simulink model "TwoArea_MA_FixedWM"  (R2020b)
settings: Solver=ode3  StartTime=0.0  StopTime=t  FixedStep=0.01  RelTol=1e-3
values from neighbouring files (symbols this model uses):
  AGC_midway = 0    [TwoAreaAGC_Parameters_Start_MA.m]    (also in result_agcimprovement.m = 1; result_replayimpact.m; result_replayimpactvaryingload.m; result_replaywithoutwm.m)
  Apc = [-par.D/(2*par.H)  1/(2*par.H)  0  -1/(2*par.H) ... (first row only)    [get_ssplant_1turb.m]
  Aq = zeros(N,N,nyp)    [offline_watermarking.m]
  attack_cont = 1    [TwoAreaAGC_Parameters_Start_MA.m]    (also in result_agcimprovement.m = 0; result_replayimpact.m; result_replayimpactvaryingload.m = 0; result_replaywithoutwm.m)
  attack_meas = 1    [TwoAreaAGC_Parameters_Start_MA.m]    (also in result_agcimprovement.m = 0; result_replayimpact.m; result_replayimpactvaryingload.m; result_replaywithoutwm.m)
  attack_start = 300    [TwoAreaAGC_Parameters_Start_MA.m]
  attack_type = 1    [TwoAreaAGC_Parameters_Start_MA.m]    (also in result_agcimprovement.m; result_replayimpact.m; result_replayimpactvaryingload.m; result_replaywithoutwm.m)
  Aw = zeros(N,N,nyp)    [offline_watermarking.m]
  Bpc = [0  -1/(2*par.H) ... (first row only)    [get_ssplant_1turb.m]
  Bq = zeros(N,1,nyp)    [offline_watermarking.m]
  Bw = zeros(N,1,nyp)    [offline_watermarking.m]
  C_sysd = c2d(C_sysc,ts_c)    [get_sscontr_2area.m]
  Cpc = [1 0 0 0 ... (first row only)    [get_ssplant_1turb.m]
  Cq = zeros(1,N,nyp)    [offline_watermarking.m]
  Cw = zeros(1,N,nyp)    [offline_watermarking.m]
  Dq = zeros(1,1,nyp)    [offline_watermarking.m]
  Dw = zeros(1,1,nyp)    [offline_watermarking.m]
  Ps = 2    [TwoAreaAGC_Parameters_Start_MA.m]
  scaling_replay = 2    [TwoAreaAGC_Parameters_Start_MA.m]    (also in result_agcimprovement.m = 1; result_replayimpact.m; result_replayimpactvaryingload.m; result_replaywithoutwm.m)
  status_load = 0    [TwoAreaAGC_Parameters_Start_MA.m]    (also in result_agcimprovement.m; result_replayimpact.m; result_replayimpactvaryingload.m = 1; result_replaywithoutwm.m)
  status_wm = 1    [TwoAreaAGC_Parameters_Start_MA.m]    (also in result_agcimprovement.m = 0; result_replayimpact.m = 0; result_replayimpactvaryingload.m = 0; result_replaywithoutwm.m = 0)
  ts = 1e-2    (= 0.01)    [TwoAreaAGC_Parameters_Start_MA.m]
undefined symbols (not defined in the file or in its folder): Ag, Ah, Bg, Bh, ca, Cg, Ch, Dg, Dh, DiscIntNeverNeededParam, Dpc, eta1, eta2, L1, L2, obs1, obs2, P1_sysd, P2_sysd, par1, par2, wm, xi1, xi2
libraries: cstblocks x16, dspsrcs4 x5, eeLuenbergerObserver x2
(part 1 of 2)
settings Model: Creator=HP  LastModifiedBy=gvandenbroek
settings DataIOCC: ReturnWorkspaceOutputs=off
settings DebuggingCC: ArithmeticOperatorsInVariantConditions=warning
settings SFSimCC: SimUseLocalCustomCode=off  CustomCodeUndefinedFunction=UseInterfaceOnly
settings RTWCC: RTWUseLocalCustomCode=off
settings CodeAppCC: StateflowObjectComments=on
settings ConfigComp: PLC_TargetIDE=twincat3

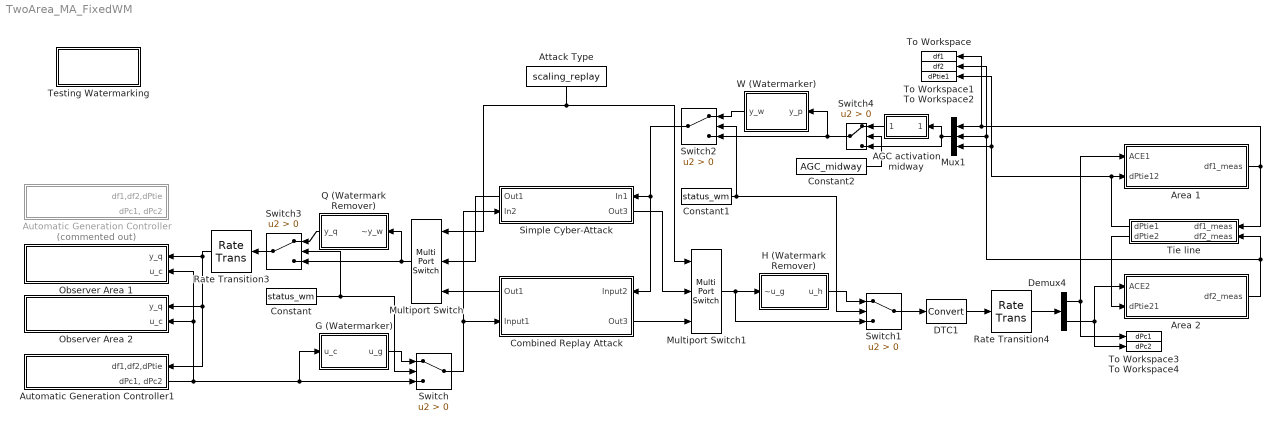
== system TwoArea_MA_FixedWM ==
  AGC activation midway : Subsystem
  Area 1 : Subsystem
  Area 2 : Subsystem
  Attack Type : Constant  Value=scaling_replay
  Automatic Generation Controller : Subsystem  Commented=on  TreatAsAtomicUnit=on
      settings: PortSchema="{\"entries\":[{\"content\":{\"sides\":[{\"content\":{\"connectorIds\":[]},\"type\":\"ConnectorPlacement.EquallySpacedRectSide\",\"uuid\":\"5549200c-2470-4b9f-b5b6-404335018806\"},{\"content\":{\"connectorIds\":[\"In1\",\"Out1\"],\"side\":\"RIGHT\"},\"type\":\"ConnectorPlacement.EquallySpacedRectSide\",\"uuid\":\"92a60021-22f8-453b-8267-494e0677e7ef\"},{\"content\":{\"connectorIds\":[],\"side\":\"TOP\"},\"type\":\"ConnectorPlacement.EquallySpacedRectSide\",\"uuid\":\"846800f7-206a-46ef-bf7f-e65eb2b7ee13\"}]},\"type\":\"ConnectorPlacement.EquallySpacedConnector\",\"uuid\":\"849222ff-13db-4c5e-adb1-95e3c523a6ec\"}],\"packageUris\":[\"http://schema.mathworks.com/mf0/Connector/19700101\"],\"version\":\"1.0\"}"
  Automatic Generation Controller1 : Subsystem  TreatAsAtomicUnit=on
      settings: PortSchema="{\"entries\":[{\"content\":{\"sides\":[{\"content\":{\"connectorIds\":[]},\"type\":\"ConnectorPlacement.EquallySpacedRectSide\",\"uuid\":\"5549200c-2470-4b9f-b5b6-404335018806\"},{\"content\":{\"connectorIds\":[\"In1\",\"Out1\"],\"side\":\"RIGHT\"},\"type\":\"ConnectorPlacement.EquallySpacedRectSide\",\"uuid\":\"92a60021-22f8-453b-8267-494e0677e7ef\"},{\"content\":{\"connectorIds\":[],\"side\":\"TOP\"},\"type\":\"ConnectorPlacement.EquallySpacedRectSide\",\"uuid\":\"846800f7-206a-46ef-bf7f-e65eb2b7ee13\"}]},\"type\":\"ConnectorPlacement.EquallySpacedConnector\",\"uuid\":\"849222ff-13db-4c5e-adb1-95e3c523a6ec\"}],\"packageUris\":[\"http://schema.mathworks.com/mf0/Connector/R2020b\"],\"version\":\"1.0\"}"
  Combined Replay Attack : Subsystem
      settings: PortSchema="{\"entries\":[{\"content\":{\"sides\":[{\"content\":{\"connectorIds\":[\"In1\",\"Out2\"]},\"type\":\"ConnectorPlacement.EquallySpacedRectSide\",\"uuid\":\"ed098d6b-24bb-4b63-8622-61583d169173\"},{\"content\":{\"connectorIds\":[\"Out1\",\"In2\"],\"side\":\"RIGHT\"},\"type\":\"ConnectorPlacement.EquallySpacedRectSide\",\"uuid\":\"5227fdb7-d0b7-460e-b294-cace27174690\"},{\"content\":{\"connectorIds\":[],\"side\":\"TOP\"},\"type\":\"ConnectorPlacement.EquallySpacedRectSide\",\"uuid\":\"40035942-24d6-4e32-87fb-1400cccdfaf4\"},{\"content\":{\"connectorIds\":[],\"side\":\"HIDDEN\"},\"type\":\"ConnectorPlacement.EquallySpacedRectSide\",\"uuid\":\"cfa004c0-44dd-4a73-bda5-a763349795eb\"}]},\"type\":\"ConnectorPlacement.EquallySpacedConnector\",\"uuid\":\"e601dc09-6e07-4799-9690-340a3e9b8374\"}],\"packageUris\":[\"http://schema.mathworks.com/mf0/Connector/R2020b\"],\"version\":\"1.0\"}"
  Constant : Constant  Value=status_wm
  Constant1 : Constant  Value=status_wm
  Constant2 : Constant  Value=AGC_midway
  DTC1 : DataTypeConversion
  Demux4 : Demux  Outputs=2
  G (Watermarker) : Subsystem
  H (Watermark Remover) : Subsystem
  Multiport Switch : MultiPortSwitch  DataPortOrder=Specify indices  DataPortIndices={1,2}
  Multiport Switch1 : MultiPortSwitch  DataPortOrder=Specify indices  DataPortIndices={1,2}
  Mux1 : Mux  Inputs=3
  Observer Area 1 : Subsystem
  Observer Area 2 : Subsystem
  Q (Watermark Remover) : Subsystem
  Rate Transition3 : RateTransition  OutPortSampleTime=ts
  Rate Transition4 : RateTransition  Integrity=off  InitialCondition=1.6  OutPortSampleTime=0
  Simple Cyber-Attack : Subsystem
      settings: PortSchema="{\"entries\":[{\"content\":{\"sides\":[{\"content\":{\"connectorIds\":[\"In1\",\"Out2\"]},\"type\":\"ConnectorPlacement.EquallySpacedRectSide\",\"uuid\":\"2958ed8f-b955-4611-80df-9c2e2faeeed8\"},{\"content\":{\"connectorIds\":[\"Out1\",\"In2\"],\"side\":\"RIGHT\"},\"type\":\"ConnectorPlacement.EquallySpacedRectSide\",\"uuid\":\"bb242c12-8aed-4e93-92e3-aa1a58434ea1\"},{\"content\":{\"connectorIds\":[],\"side\":\"TOP\"},\"type\":\"ConnectorPlacement.EquallySpacedRectSide\",\"uuid\":\"026445f8-91a1-47c1-afd6-e1ddb7405b1a\"},{\"content\":{\"connectorIds\":[],\"side\":\"BOTTOM\"},\"type\":\"ConnectorPlacement.EquallySpacedRectSide\",\"uuid\":\"f5ef18f8-9aaf-4c82-8169-2595013f0f61\"}]},\"type\":\"ConnectorPlacement.EquallySpacedConnector\",\"uuid\":\"16e2adc2-f66f-41a6-a84c-2e0eb9d1d8a6\"}],\"packageUris\":[\"http://schema.mathworks.com/mf0/Connector/19700101\"],\"version\":\"1.0\"}"
  Switch{,1..4} (5 alike) : Switch  Criteria=u2 > Threshold
  Testing Watermarking : Subsystem
  Tie line : Subsystem
  To Workspace : ToWorkspace  VariableName=df1  SampleTime=ts
  To Workspace1 : ToWorkspace  VariableName=df2  SampleTime=ts
  To Workspace2 : ToWorkspace  VariableName=dPtie1  SampleTime=ts
  To Workspace3 : ToWorkspace  VariableName=dPc1  SampleTime=ts
  To Workspace4 : ToWorkspace  VariableName=dPc2  SampleTime=ts
  W (Watermarker) : Subsystem  TreatAsAtomicUnit=on
  wires:
  Attack Type/1 -> Multiport Switch1/1, Multiport Switch/1
  Simple Cyber-Attack/1(Out1) -> Multiport Switch/2
  Switch3/1 -> Rate Transition3/1
  DTC1/1 -> Rate Transition4/1
  Multiport Switch/1 -> Switch3/3, Q (Watermark Remover)/1(~y_w)
  W (Watermarker)/1(y_w) -> Switch2/1
  Switch2/1 -> Combined Replay Attack/1(Input2), Simple Cyber-Attack/1(In1)
  Rate Transition3/1 -> Automatic Generation Controller1/1(df1,df2,dPtie), Observer Area 2/1(y_q), Observer Area 1/1(y_q)
  Q (Watermark Remover)/1(y_q) -> Switch3/1
  Simple Cyber-Attack/2(Out3) -> Multiport Switch1/2
  H (Watermark Remover)/1(u_h) -> Switch1/1
  Switch/1 -> Simple Cyber-Attack/2(In2), Combined Replay Attack/2(Input1)
  G (Watermarker)/1(u_g) -> Switch/1
  Switch1/1 -> DTC1/1
  Multiport Switch1/1 -> Switch1/3, H (Watermark Remover)/1(~u_g)
  Area 1/1(df1_meas) -> To Workspace/1, Mux1/1, Tie line/1(df1_meas)
  Area 2/1(df2_meas) -> To Workspace1/1, Mux1/2, Tie line/2(df2_meas)
  Tie line/2(dPtie2) -> Area 2/2(dPtie21)
  Tie line/1(dPtie1) -> To Workspace2/1, Mux1/3, Area 1/2(dPtie12)
  Automatic Generation Controller1/1("dPc1, dPc2") -> Observer Area 2/2(u_c), Observer Area 1/2(u_c), Switch/3, G (Watermarker)/1(u_c)
  Demux4/1 -> To Workspace3/1, Area 1/1(ACE1)
  Demux4/2 -> To Workspace4/1, Area 2/1(ACE2)
  Rate Transition4/1 -> Demux4/1
  Switch4/1 -> Switch2/3, W (Watermarker)/1(y_p)
  Constant/1 -> Switch/2, Switch3/2
  Constant1/1 -> Switch2/2, Switch1/2
  AGC activation midway/1(Out1) -> Switch4/1
  Mux1/1 -> Switch4/3, AGC activation midway/1(In1)
  Constant2/1 -> Switch4/2
  Combined Replay Attack/1(Out1) -> Multiport Switch/3
  Combined Replay Attack/2(Out3) -> Multiport Switch1/3

== system TwoArea_MA_FixedWM/AGC activation midway ==
  In1 : Inport
  Clock : Clock
  Constant : Constant  Value=0
  Demux : Demux  Outputs=3
  Mux : Mux  Inputs=3
  Switch : Switch  Threshold=attack_start
  Switch1 : Switch  Threshold=attack_start
  Switch2 : Switch  Threshold=attack_start
  Out1 : Outport
  wires:
  Switch/1 -> Mux/1
  Clock/1 -> Switch2/2, Switch1/2, Switch/2
  Demux/1 -> Switch/1
  Constant/1 -> Switch2/3, Switch1/3, Switch/3
  Demux/2 -> Switch1/1
  Switch1/1 -> Mux/2
  Demux/3 -> Switch2/1
  Switch2/1 -> Mux/3
  Mux/1 -> Out1/1
  In1/1 -> Demux/1

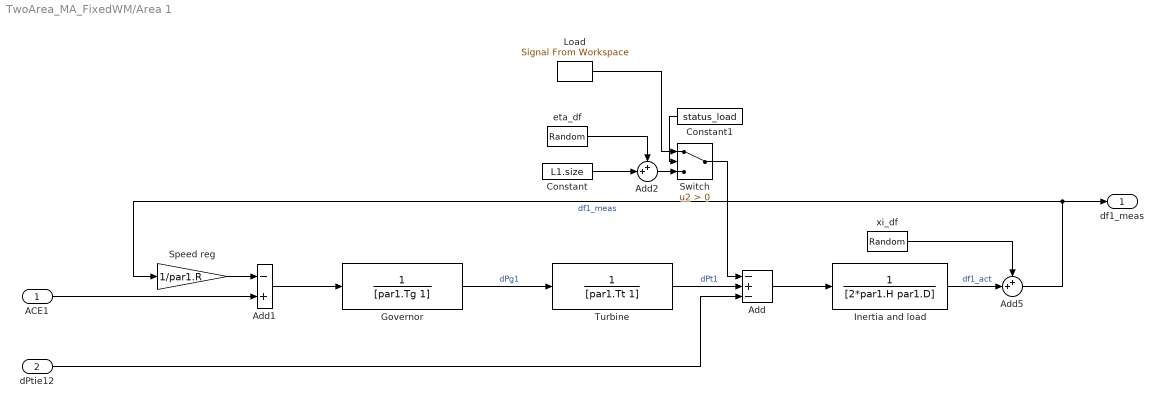
== system TwoArea_MA_FixedWM/Area 1 ==
  ACE1 : Inport
  dPtie12 : Inport  Port=2
  Add : Sum  Inputs=-+-
  Add1 : Sum  Inputs=-+
  Add2 : Sum  Inputs=++|
  Add5 : Sum  Inputs=++|
  Constant : Constant  Value=L1.size
  Constant1 : Constant  Value=status_load
  Governor : TransferFcn  Denominator=[par1.Tg 1]
  Inertia and load : TransferFcn  Denominator=[2*par1.H par1.D]
  Load : dspsrcs4/Signal From Workspace  X=L1.seq  Ts=1  nsamps=1  OutputAfterFinalValue=Holding final value  ignoreOrWarnInputAndFrameLengths=off  OutputFrames=off
  Speed reg : Gain  Gain=1/par1.R
  Switch : Switch  Criteria=u2 > Threshold
  Turbine : TransferFcn  Denominator=[par1.Tt 1]
  eta_df : RandomNumber  Variance=eta1.var(1)  Seed=eta1.seeddf  SampleTime=0
  xi_df : RandomNumber  Variance=xi1.var(1)  Seed=xi1.seeddf  SampleTime=0
  df1_meas : Outport
  wires:
  xi_df/1 -> Add5/1
  Add/1 -> Inertia and load/1
  Governor/1 -> Turbine/1  "dPg1"
  Turbine/1 -> Add/2  "dPt1"
  ACE1/1 -> Add1/2
  Add5/1 -> Speed reg/1, df1_meas/1  "df1_meas"
  Add1/1 -> Governor/1
  Inertia and load/1 -> Add5/2  "df1_act"
  Speed reg/1 -> Add1/1
  dPtie12/1 -> Add/3
  Constant/1 -> Add2/2
  eta_df/1 -> Add2/1
  Add2/1 -> Switch/3
  Switch/1 -> Add/1
  Load/1 -> Switch/1
  Constant1/1 -> Switch/2

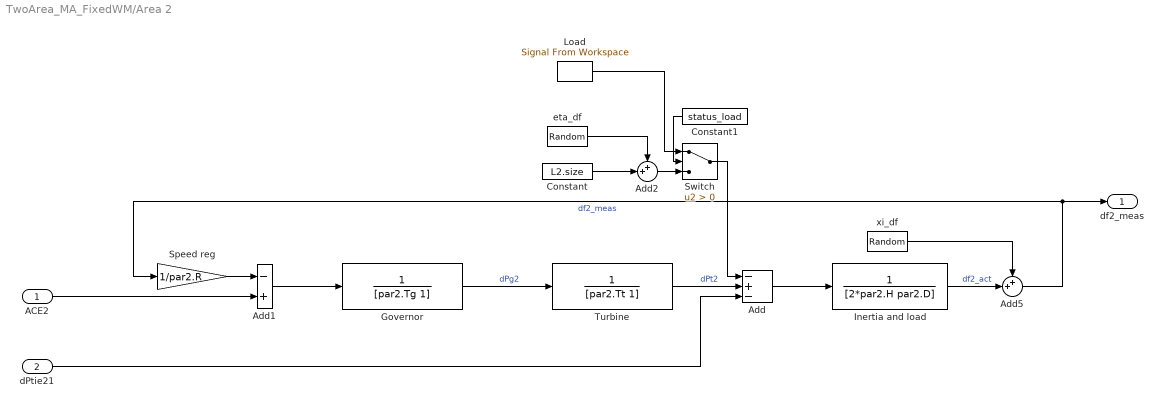
== system TwoArea_MA_FixedWM/Area 2 ==
  ACE2 : Inport
  dPtie21 : Inport  Port=2
  Add : Sum  Inputs=-+-
  Add1 : Sum  Inputs=-+
  Add2 : Sum  Inputs=++|
  Add5 : Sum  Inputs=++|
  Constant : Constant  Value=L2.size
  Constant1 : Constant  Value=status_load
  Governor : TransferFcn  Denominator=[par2.Tg 1]
  Inertia and load : TransferFcn  Denominator=[2*par2.H par2.D]
  Load : dspsrcs4/Signal From Workspace  X=L2.seq  Ts=1  nsamps=1  OutputAfterFinalValue=Holding final value  ignoreOrWarnInputAndFrameLengths=off  OutputFrames=off
  Speed reg : Gain  Gain=1/par2.R
  Switch : Switch  Criteria=u2 > Threshold
  Turbine : TransferFcn  Denominator=[par2.Tt 1]
  eta_df : RandomNumber  Variance=eta2.var(1)  Seed=eta1.seeddf  SampleTime=0
  xi_df : RandomNumber  Variance=xi2.var(1)  Seed=xi2.seeddf  SampleTime=0
  df2_meas : Outport
  wires:
  xi_df/1 -> Add5/1
  Add/1 -> Inertia and load/1
  Governor/1 -> Turbine/1  "dPg2"
  Turbine/1 -> Add/2  "dPt2"
  ACE2/1 -> Add1/2
  Add5/1 -> Speed reg/1, df2_meas/1  "df2_meas"
  Add1/1 -> Governor/1
  Inertia and load/1 -> Add5/2  "df2_act"
  Speed reg/1 -> Add1/1
  dPtie21/1 -> Add/3
  Constant/1 -> Add2/2
  eta_df/1 -> Add2/1
  Switch/1 -> Add/1
  Load/1 -> Switch/1
  Add2/1 -> Switch/3
  Constant1/1 -> Switch/2

== system TwoArea_MA_FixedWM/Automatic Generation Controller ==
  df1,df2,dPtie : Inport
  DTC5 : DataTypeConversion
  Discrete State-Space : DiscreteStateSpace  A=C_sysd.A  B=C_sysd.B  C=C_sysd.C  D=C_sysd.D  InitialCondition=[0 0]  SampleTime=-1
  Rate Transition1 : RateTransition  Integrity=off  InitialCondition=1.6  OutPortSampleTime=ts
  Rate Transition2 : RateTransition  OutPortSampleTime=ts_c
  "dPc1, dPc2" : Outport
  wires:
  Rate Transition2/1 -> Discrete State-Space/1
  DTC5/1 -> Rate Transition1/1
  Rate Transition1/1 -> "dPc1, dPc2"/1
  df1,df2,dPtie/1 -> Rate Transition2/1
  Discrete State-Space/1 -> DTC5/1

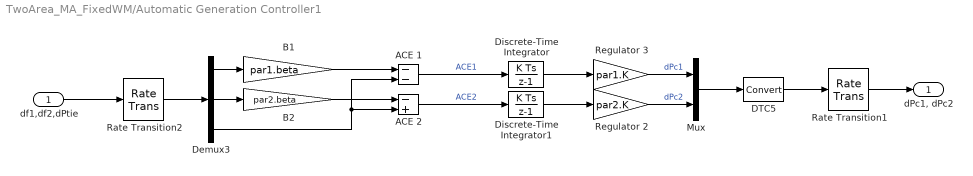
== system TwoArea_MA_FixedWM/Automatic Generation Controller1 ==
  df1,df2,dPtie : Inport
  ACE 1 : Sum  Inputs=--
  ACE 2 : Sum  Inputs=-+
  B1 : Gain  Gain=par1.beta
  B2 : Gain  Gain=par2.beta
  DTC5 : DataTypeConversion
  Demux3 : Demux  Outputs=3
  Discrete-Time Integrator : DiscreteIntegrator  SampleTime=2  ICPrevOutput=DiscIntNeverNeededParam  ICPrevScaledInput=DiscIntNeverNeededParam
  Discrete-Time Integrator1 : DiscreteIntegrator  SampleTime=2  ICPrevOutput=DiscIntNeverNeededParam  ICPrevScaledInput=DiscIntNeverNeededParam
  Mux : Mux  Inputs=2
  Rate Transition1 : RateTransition  Integrity=off  InitialCondition=1.6  OutPortSampleTime=ts
  Rate Transition2 : RateTransition  OutPortSampleTime=ts_c
  Regulator 2 : Gain  Gain=par2.K
  Regulator 3 : Gain  Gain=par1.K
  "dPc1, dPc2" : Outport
  wires:
  Demux3/2 -> B2/1
  Demux3/3 -> ACE 2/2, ACE 1/2
  Mux/1 -> DTC5/1
  Rate Transition2/1 -> Demux3/1
  Demux3/1 -> B1/1
  ACE 2/1 -> Discrete-Time Integrator1/1  "ACE2"
  DTC5/1 -> Rate Transition1/1
  Regulator 3/1 -> Mux/1  "dPc1"
  ACE 1/1 -> Discrete-Time Integrator/1  "ACE1"
  Discrete-Time Integrator/1 -> Regulator 3/1
  B1/1 -> ACE 1/1
  Regulator 2/1 -> Mux/2  "dPc2"
  B2/1 -> ACE 2/1
  Discrete-Time Integrator1/1 -> Regulator 2/1
  Rate Transition1/1 -> "dPc1, dPc2"/1
  df1,df2,dPtie/1 -> Rate Transition2/1

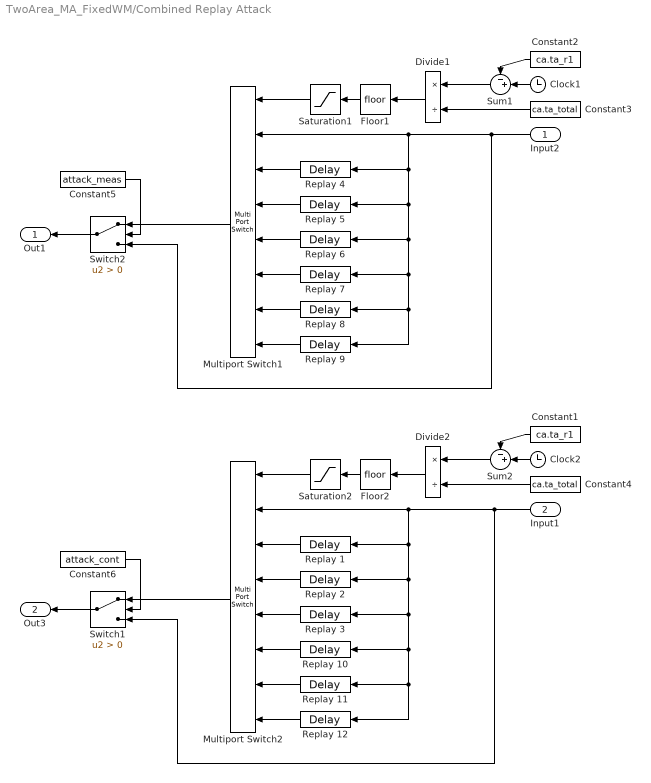
== system TwoArea_MA_FixedWM/Combined Replay Attack ==
  Input2 : Inport
  Input1 : Inport  Port=2
  Clock1 : Clock
  Clock2 : Clock
  Constant1 : Constant  Value=ca.ta_r1
  Constant2 : Constant  Value=ca.ta_r1
  Constant3 : Constant  Value=ca.ta_total
  Constant4 : Constant  Value=ca.ta_total
  Constant5 : Constant  Value=attack_meas
  Constant6 : Constant  Value=attack_cont
  Divide1 : Product  Inputs=*/  OutMin=0  OutMax=3  SaturateOnIntegerOverflow=on
  Divide2 : Product  Inputs=*/  OutMin=0  OutMax=3  SaturateOnIntegerOverflow=on
  Floor1 : Rounding
  Floor2 : Rounding
  Multiport Switch1 : MultiPortSwitch  DataPortOrder=Zero-based contiguous  Inputs=7  zeroidx=on
  Multiport Switch2 : MultiPortSwitch  DataPortOrder=Zero-based contiguous  Inputs=7  zeroidx=on
  Replay 1 : TransportDelay  DelayTime=ca.ta_total
  Replay 10 : TransportDelay  DelayTime=ca.ta_total*4
  Replay 11 : TransportDelay  DelayTime=ca.ta_total*5
  Replay 12 : TransportDelay  DelayTime=ca.ta_total*6
  Replay 2 : TransportDelay  DelayTime=ca.ta_total*2
  Replay 3 : TransportDelay  DelayTime=ca.ta_total*3
  Replay 4 : TransportDelay  DelayTime=ca.ta_total
  Replay 5 : TransportDelay  DelayTime=ca.ta_total*2
  Replay 6 : TransportDelay  DelayTime=ca.ta_total*3
  Replay 7 : TransportDelay  DelayTime=ca.ta_total*4
  Replay 8 : TransportDelay  DelayTime=ca.ta_total*5
  Replay 9 : TransportDelay  DelayTime=ca.ta_total*6
  Saturation1 : Saturate  UpperLimit=6  LowerLimit=0
  Saturation2 : Saturate  UpperLimit=6  LowerLimit=0
  Sum1 : Sum  Inputs=-+|
  Sum2 : Sum  Inputs=-+|
  Switch1 : Switch  Criteria=u2 > Threshold
  Switch2 : Switch  Criteria=u2 > Threshold
  Out1 : Outport
  Out3 : Outport  Port=2
  wires:
  Replay 6/1 -> Multiport Switch1/5
  Sum1/1 -> Divide1/1
  Replay 4/1 -> Multiport Switch1/3
  Multiport Switch1/1 -> Switch2/1
  Clock1/1 -> Sum1/2
  Saturation1/1 -> Multiport Switch1/1
  Input2/1 -> Switch2/3, Replay 9/1, Replay 8/1, Replay 7/1, Replay 6/1, Replay 5/1, Replay 4/1, Multiport Switch1/2
  Constant3/1 -> Divide1/2
  Floor1/1 -> Saturation1/1
  Constant2/1 -> Sum1/1
  Replay 5/1 -> Multiport Switch1/4
  Divide1/1 -> Floor1/1
  Replay 9/1 -> Multiport Switch1/8
  Replay 8/1 -> Multiport Switch1/7
  Replay 7/1 -> Multiport Switch1/6
  Replay 10/1 -> Multiport Switch2/6
  Replay 11/1 -> Multiport Switch2/7
  Replay 12/1 -> Multiport Switch2/8
  Divide2/1 -> Floor2/1
  Clock2/1 -> Sum2/2
  Constant1/1 -> Sum2/1
  Replay 2/1 -> Multiport Switch2/4
  Multiport Switch2/1 -> Switch1/1
  Constant4/1 -> Divide2/2
  Replay 3/1 -> Multiport Switch2/5
  Floor2/1 -> Saturation2/1
  Input1/1 -> Switch1/3, Replay 12/1, Replay 11/1, Replay 10/1, Replay 3/1, Replay 2/1, Replay 1/1, Multiport Switch2/2
  Sum2/1 -> Divide2/1
  Saturation2/1 -> Multiport Switch2/1
  Replay 1/1 -> Multiport Switch2/3
  Switch2/1 -> Out1/1
  Switch1/1 -> Out3/1
  Constant5/1 -> Switch2/2
  Constant6/1 -> Switch1/2

== system TwoArea_MA_FixedWM/G (Watermarker) ==
  u_c : Inport
  " G selector" : Subsystem
  " G selector1" : Subsystem
  Demux1 : Demux  Outputs=2
  Discrete Varying State Space3 : cstblocks/Linear Parameter Varying/Discrete Varying State Space  x0=zeros(wm.N,1)  Ts=ts  OutputX=off  OutputDX=off
      settings: SourceProductBaseCode=CT
  Discrete Varying State Space4 : cstblocks/Linear Parameter Varying/Discrete Varying State Space  x0=zeros(wm.N,1)  Ts=ts  OutputX=off  OutputDX=off
      settings: SourceProductBaseCode=CT
  Mux3 : Mux  Inputs=2
  u_g : Outport
  wires:
  " G selector1"/2(Bg) -> Discrete Varying State Space3/3
  " G selector"/3(Cg) -> Discrete Varying State Space4/4
  " G selector1"/3(Cg) -> Discrete Varying State Space3/4
  Discrete Varying State Space3/1 -> Mux3/2
  " G selector"/2(Bg) -> Discrete Varying State Space4/3
  Discrete Varying State Space4/1 -> Mux3/1
  " G selector"/1(Ag) -> Discrete Varying State Space4/2
  " G selector1"/1(Ag) -> Discrete Varying State Space3/2
  " G selector1"/4(Dg) -> Discrete Varying State Space3/5
  Demux1/1 -> Discrete Varying State Space4/1
  Demux1/2 -> Discrete Varying State Space3/1
  " G selector"/4(Dg) -> Discrete Varying State Space4/5
  u_c/1 -> Demux1/1
  Mux3/1 -> u_g/1

== system TwoArea_MA_FixedWM/H (Watermark Remover) ==
  ~u_g : Inport
  " H selector" : Subsystem
  " H selector1" : Subsystem
  Demux1 : Demux  Outputs=2
  Discrete Varying State Space3 : cstblocks/Linear Parameter Varying/Discrete Varying State Space  x0=zeros(wm.N,1)  Ts=ts  OutputX=off  OutputDX=off
      settings: SourceProductBaseCode=CT
  Discrete Varying State Space4 : cstblocks/Linear Parameter Varying/Discrete Varying State Space  x0=zeros(wm.N,1)  Ts=ts  OutputX=off  OutputDX=off
      settings: SourceProductBaseCode=CT
  Mux3 : Mux  Inputs=2
  u_h : Outport
  wires:
  " H selector1"/2(Bh) -> Discrete Varying State Space3/3
  " H selector"/3(Ch) -> Discrete Varying State Space4/4
  " H selector1"/3(Ch) -> Discrete Varying State Space3/4
  Discrete Varying State Space3/1 -> Mux3/2
  " H selector"/2(Bh) -> Discrete Varying State Space4/3
  Discrete Varying State Space4/1 -> Mux3/1
  " H selector"/1(Ah) -> Discrete Varying State Space4/2
  " H selector1"/1(Ah) -> Discrete Varying State Space3/2
  " H selector1"/4(Dh) -> Discrete Varying State Space3/5
  Demux1/1 -> Discrete Varying State Space4/1
  Demux1/2 -> Discrete Varying State Space3/1
  " H selector"/4(Dh) -> Discrete Varying State Space4/5
  ~u_g/1 -> Demux1/1
  Mux3/1 -> u_h/1

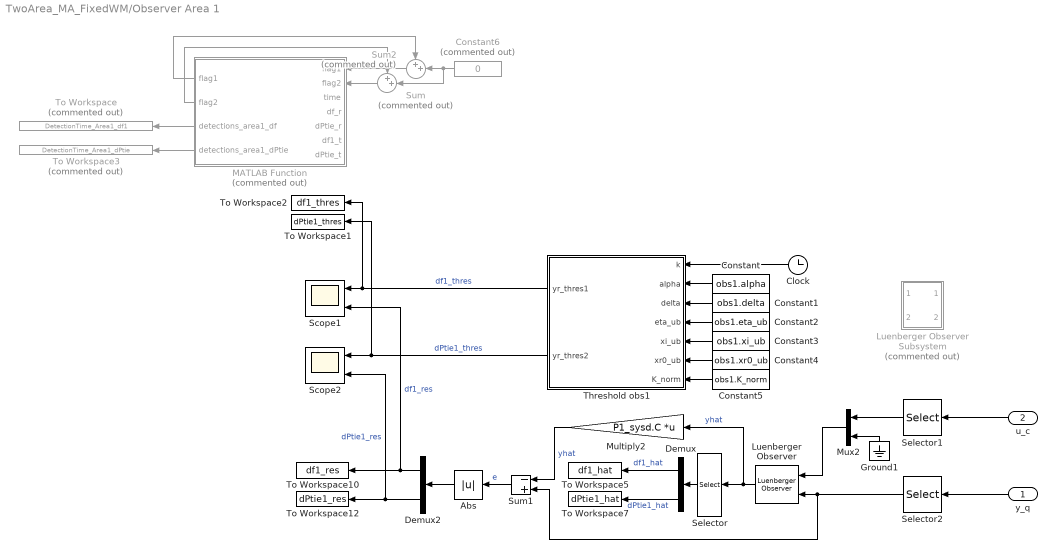
== system TwoArea_MA_FixedWM/Observer Area 1 ==
  y_q : Inport
  u_c : Inport  Port=2
  Abs : Abs  ZeroCross=off
  Clock : Clock
  Constant : Constant  Value=obs1.alpha
  Constant1 : Constant  Value=obs1.delta
  Constant2 : Constant  Value=obs1.eta_ub
  Constant3 : Constant  Value=obs1.xi_ub
  Constant4 : Constant  Value=obs1.xr0_ub
  Constant5 : Constant  Value=obs1.K_norm
  Constant6 : Constant  Commented=on  Value=0
  Demux : Demux  Outputs=2
  Demux2 : Demux  Outputs=2
  Ground1 : Ground
  Luenberger Observer Subsystem : Subsystem  Commented=on  TreatAsAtomicUnit=on
  Luenberger Observer : eeLuenbergerObserver/Luenberger Observer  StateSpaceType=Discrete-time  Ad=P1_sysd.A  Bd=P1_sysd.B  Cd=P1_sysd.C  Dd=P1_sysd.D  A=Apc  B=Bpc  C=Cpc  D=Dpc  ObserverDesign=Observer gain  Ld=obs1.K  DesiredEigenvalues=poles  x0=obs1.x_hat0  Tsd=ts  Ts=ts
      settings: SourceProductBaseCode=PS
  MATLAB Function : MATLAB Function  Commented=on  TreatAsAtomicUnit=on
  Multiply2 : Gain  Gain=P1_sysd.C  Multiplication=Matrix(K*u)
  Mux2 : Mux  Inputs=2
  Scope1 : Scope  NumInputPorts=2
  Scope2 : Scope  NumInputPorts=2
  Selector : Selector  InputPortWidth=4  IndexOptions=Index vector (dialog)  Indices=[1 4 ]  OutputSizes=1
  Selector1 : Selector  InputPortWidth=2  IndexOptions=Index vector (dialog)  Indices=1  OutputSizes=1
  Selector2 : Selector  InputPortWidth=3  IndexOptions=Index vector (dialog)  Indices=[1 3]  OutputSizes=1
  Sum : Sum  Commented=on  Inputs=++|
  Sum1 : Sum  Inputs=-+
  Sum2 : Sum  Commented=on  Inputs=++|
  Threshold obs1 : MATLAB Function  TreatAsAtomicUnit=on
  To Workspace : ToWorkspace  Commented=on  VariableName=DetectionTime_Area1_df1  SampleTime=-1
  To Workspace1 : ToWorkspace  VariableName=dPtie1_thres  SampleTime=ts
  To Workspace10 : ToWorkspace  VariableName=df1_res  SampleTime=ts
  To Workspace12 : ToWorkspace  VariableName=dPtie1_res  SampleTime=ts
  To Workspace2 : ToWorkspace  VariableName=df1_thres  SampleTime=ts
  To Workspace3 : ToWorkspace  Commented=on  VariableName=DetectionTime_Area1_dPtie  SampleTime=-1
  To Workspace5 : ToWorkspace  VariableName=df1_hat  SampleTime=ts
  To Workspace7 : ToWorkspace  VariableName=dPtie1_hat  SampleTime=ts
  wires:
  Sum1/1 -> Abs/1  "e"
  Selector2/1 -> Luenberger Observer/2, Sum1/2
  Selector/1 -> Demux/1
  Demux2/1 -> To Workspace10/1, Scope1/2  "df1_res"
  Constant4/1 -> Threshold obs1/6(xr0_ub)
  Demux2/2 -> To Workspace12/1, Scope2/2  "dPtie1_res"
  Ground1/1 -> Mux2/2
  Abs/1 -> Demux2/1
  Constant3/1 -> Threshold obs1/5(xi_ub)
  Luenberger Observer/1 -> Multiply2/1, Selector/1  "yhat"
  Constant1/1 -> Threshold obs1/3(delta)
  Threshold obs1/1(yr_thres1) -> To Workspace2/1, Scope1/1  "df1_thres"
  Clock/1 -> Threshold obs1/1(k)
  Demux/1 -> To Workspace5/1  "df1_hat"
  Constant2/1 -> Threshold obs1/4(eta_ub)
  Constant5/1 -> Threshold obs1/7(K_norm)
  Constant/1 -> Threshold obs1/2(alpha)
  Selector1/1 -> Mux2/1
  Demux/2 -> To Workspace7/1  "dPtie1_hat"
  Threshold obs1/2(yr_thres2) -> To Workspace1/1, Scope2/1  "dPtie1_thres"
  y_q/1 -> Selector2/1
  u_c/1 -> Selector1/1
  Mux2/1 -> Luenberger Observer/1
  Multiply2/1 -> Sum1/1  "yhat"
  Constant6/1 -> Sum2/2, Sum/2
  Sum/1 -> MATLAB Function/1("flag1 ")
  Sum2/1 -> MATLAB Function/2("flag2 ")
  MATLAB Function/1(flag1) -> Sum/1
  MATLAB Function/2(flag2) -> Sum2/1
  MATLAB Function/3(detections_area1_df) -> To Workspace/1
  MATLAB Function/4(detections_area1_dPtie) -> To Workspace3/1

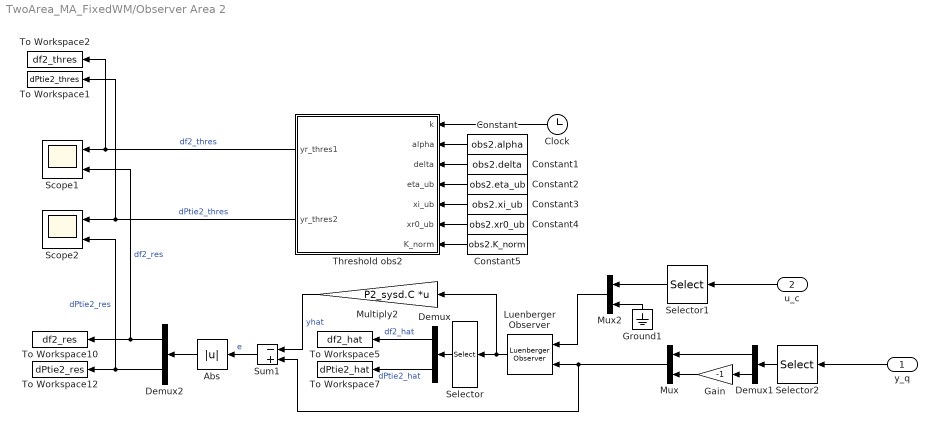
== system TwoArea_MA_FixedWM/Observer Area 2 ==
  y_q : Inport
  u_c : Inport  Port=2
  Abs : Abs  ZeroCross=off
  Clock : Clock
  Constant : Constant  Value=obs2.alpha
  Constant1 : Constant  Value=obs2.delta
  Constant2 : Constant  Value=obs2.eta_ub
  Constant3 : Constant  Value=obs2.xi_ub
  Constant4 : Constant  Value=obs2.xr0_ub
  Constant5 : Constant  Value=obs2.K_norm
  Demux : Demux  Outputs=2
  Demux1 : Demux  Outputs=2
  Demux2 : Demux  Outputs=2
  Gain : Gain  Gain=-1
  Ground1 : Ground
  Luenberger Observer : eeLuenbergerObserver/Luenberger Observer  StateSpaceType=Discrete-time  Ad=P2_sysd.A  Bd=P2_sysd.B  Cd=P2_sysd.C  Dd=P2_sysd.D  A=Apc  B=Bpc  C=Cpc  D=Dpc  ObserverDesign=Observer gain  Ld=obs2.K  DesiredEigenvalues=poles  x0=obs2.x_hat0  Tsd=ts  Ts=ts
      settings: SourceProductBaseCode=PS
  Multiply2 : Gain  Gain=P2_sysd.C  Multiplication=Matrix(K*u)
  Mux : Mux  Inputs=2
  Mux2 : Mux  Inputs=2
  Scope1 : Scope  NumInputPorts=2
  Scope2 : Scope  NumInputPorts=2
  Selector : Selector  InputPortWidth=4  IndexOptions=Index vector (dialog)  Indices=[1 4 ]  OutputSizes=1
  Selector1 : Selector  InputPortWidth=2  IndexOptions=Index vector (dialog)  Indices=2  OutputSizes=1
  Selector2 : Selector  InputPortWidth=3  IndexOptions=Index vector (dialog)  Indices=[2 3]  OutputSizes=1
  Sum1 : Sum  Inputs=-+
  Threshold obs2 : MATLAB Function  TreatAsAtomicUnit=on
  To Workspace1 : ToWorkspace  VariableName=dPtie2_thres  SampleTime=ts
  To Workspace10 : ToWorkspace  VariableName=df2_res  SampleTime=ts
  To Workspace12 : ToWorkspace  VariableName=dPtie2_res  SampleTime=ts
  To Workspace2 : ToWorkspace  VariableName=df2_thres  SampleTime=ts
  To Workspace5 : ToWorkspace  VariableName=df2_hat  SampleTime=ts
  To Workspace7 : ToWorkspace  VariableName=dPtie2_hat  SampleTime=ts
  wires:
  Sum1/1 -> Abs/1  "e"
  Selector/1 -> Demux/1
  Demux2/1 -> Scope1/2, To Workspace10/1  "df2_res"
  Luenberger Observer/1 -> Multiply2/1, Selector/1
  Constant4/1 -> Threshold obs2/6(xr0_ub)
  Demux2/2 -> Scope2/2, To Workspace12/1  "dPtie2_res"
  Ground1/1 -> Mux2/2
  Abs/1 -> Demux2/1
  Mux2/1 -> Luenberger Observer/1
  Constant3/1 -> Threshold obs2/5(xi_ub)
  Multiply2/1 -> Sum1/1  "yhat"
  Constant1/1 -> Threshold obs2/3(delta)
  Threshold obs2/1(yr_thres1) -> To Workspace2/1, Scope1/1  "df2_thres"
  Clock/1 -> Threshold obs2/1(k)
  Demux/1 -> To Workspace5/1  "df2_hat"
  Constant2/1 -> Threshold obs2/4(eta_ub)
  Constant5/1 -> Threshold obs2/7(K_norm)
  Constant/1 -> Threshold obs2/2(alpha)
  Selector1/1 -> Mux2/1
  Demux/2 -> To Workspace7/1  "dPtie2_hat"
  Threshold obs2/2(yr_thres2) -> To Workspace1/1, Scope2/1  "dPtie2_thres"
  y_q/1 -> Selector2/1
  u_c/1 -> Selector1/1
  Selector2/1 -> Demux1/1
  Demux1/2 -> Gain/1
  Gain/1 -> Mux/2
  Demux1/1 -> Mux/1
  Mux/1 -> Sum1/2, Luenberger Observer/2

== system TwoArea_MA_FixedWM/Q (Watermark Remover) ==
  ~y_w : Inport
  " Q selector" : Subsystem
  " Q selector1" : Subsystem
  " Q selector2" : Subsystem
  Demux1 : Demux  Outputs=3
  Discrete Varying State Space1 : cstblocks/Linear Parameter Varying/Discrete Varying State Space  x0=zeros(wm.N,1)  Ts=ts  OutputX=off  OutputDX=off
      settings: SourceProductBaseCode=CT
  Discrete Varying State Space3 : cstblocks/Linear Parameter Varying/Discrete Varying State Space  x0=zeros(wm.N,1)  Ts=ts  OutputX=off  OutputDX=off
      settings: SourceProductBaseCode=CT
  Discrete Varying State Space4 : cstblocks/Linear Parameter Varying/Discrete Varying State Space  x0=zeros(wm.N,1)  Ts=ts  OutputX=off  OutputDX=off
      settings: SourceProductBaseCode=CT
  Mux3 : Mux  Inputs=3
  y_q : Outport
  wires:
  " Q selector"/3(Cq) -> Discrete Varying State Space4/4
  " Q selector2"/2(Bq) -> Discrete Varying State Space1/3
  Discrete Varying State Space1/1 -> Mux3/3
  Discrete Varying State Space3/1 -> Mux3/2
  " Q selector"/2(Bq) -> Discrete Varying State Space4/3
  Discrete Varying State Space4/1 -> Mux3/1
  " Q selector"/1(Aq) -> Discrete Varying State Space4/2
  " Q selector2"/4(Dq) -> Discrete Varying State Space1/5
  " Q selector2"/1(Aq) -> Discrete Varying State Space1/2
  " Q selector2"/3(Cq) -> Discrete Varying State Space1/4
  Demux1/1 -> Discrete Varying State Space4/1
  Demux1/3 -> Discrete Varying State Space1/1
  Demux1/2 -> Discrete Varying State Space3/1
  " Q selector"/4(Dq) -> Discrete Varying State Space4/5
  ~y_w/1 -> Demux1/1
  Mux3/1 -> y_q/1
  " Q selector1"/1(Aq) -> Discrete Varying State Space3/2
  " Q selector1"/2(Bq) -> Discrete Varying State Space3/3
  " Q selector1"/3(Cq) -> Discrete Varying State Space3/4
  " Q selector1"/4(Dq) -> Discrete Varying State Space3/5

== system TwoArea_MA_FixedWM/Simple Cyber-Attack ==
  In1 : Inport
  In2 : Inport  Port=2
  Constant1 : Constant  Value=attack_meas
  Constant2 : Constant  Value=attack_cont
  Cyber-attack control commands : Subsystem
  Cyber-attack measurements : Subsystem
  Switch1 : Switch  Criteria=u2 > Threshold
  Switch2 : Switch  Criteria=u2 > Threshold
  Out1 : Outport
  Out3 : Outport  Port=2
  wires:
  In2/1 -> Switch1/3, Cyber-attack control commands/1(In1)
  Switch2/1 -> Out1/1
  In1/1 -> Switch2/3, Cyber-attack measurements/1(In1)
  Switch1/1 -> Out3/1
  Constant1/1 -> Switch2/2
  Constant2/1 -> Switch1/2
  Cyber-attack measurements/1(Out1) -> Switch2/1
  Cyber-attack control commands/1(Out1) -> Switch1/1

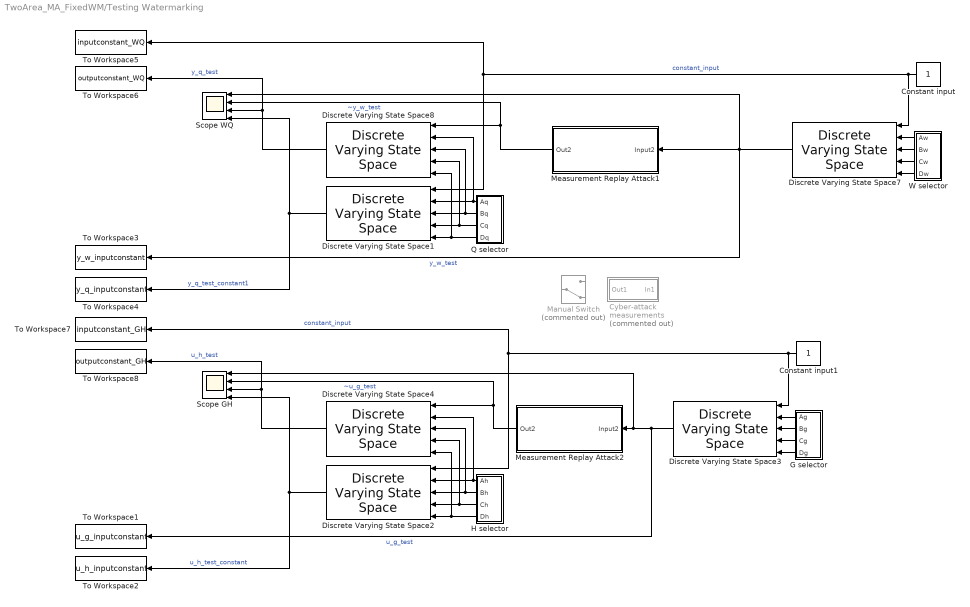
== system TwoArea_MA_FixedWM/Testing Watermarking ==
  " G selector" : Subsystem
  " H selector" : Subsystem
  " Q selector" : Subsystem
  " W selector" : Subsystem
  Constant input : Constant
  Constant input1 : Constant
  Cyber-attack measurements : Subsystem  Commented=on
  Discrete Varying State Space{1..4,7..8} (6 alike) : cstblocks/Linear Parameter Varying/Discrete Varying State Space  x0=zeros(wm.N,1)  Ts=ts  OutputX=off  OutputDX=off
      settings: SourceProductBaseCode=CT
  Manual Switch : ManualSwitch  Commented=on  CurrentSetting=0
  Measurement Replay Attack1 : Subsystem
  Measurement Replay Attack2 : Subsystem
  Scope GH : Scope  NumInputPorts=4
  Scope WQ : Scope  NumInputPorts=4
  To Workspace1 : ToWorkspace  VariableName=u_g_inputconstant  SampleTime=ts
  To Workspace2 : ToWorkspace  VariableName=u_h_inputconstant  SampleTime=ts
  To Workspace3 : ToWorkspace  VariableName=y_w_inputconstant  SampleTime=ts
  To Workspace4 : ToWorkspace  VariableName=y_q_inputconstant  SampleTime=ts
  To Workspace5 : ToWorkspace  VariableName=inputconstant_WQ  SampleTime=ts
  To Workspace6 : ToWorkspace  VariableName=outputconstant_WQ  SampleTime=ts
  To Workspace7 : ToWorkspace  VariableName=inputconstant_GH  SampleTime=ts
  To Workspace8 : ToWorkspace  VariableName=outputconstant_GH  SampleTime=ts
  wires:
  " Q selector"/4(Dq) -> Discrete Varying State Space8/5, Discrete Varying State Space1/5
  " Q selector"/2(Bq) -> Discrete Varying State Space8/3, Discrete Varying State Space1/3
  " Q selector"/3(Cq) -> Discrete Varying State Space8/4, Discrete Varying State Space1/4
  Discrete Varying State Space7/1 -> Measurement Replay Attack1/1(Input2), Scope WQ/1, To Workspace3/1  "y_w_test"
  Discrete Varying State Space8/1 -> To Workspace6/1, Scope WQ/3  "y_q_test"
  Constant input/1 -> Discrete Varying State Space7/1, Discrete Varying State Space1/1, To Workspace5/1  "constant_input"
  " W selector"/3(Cw) -> Discrete Varying State Space7/4
  " Q selector"/1(Aq) -> Discrete Varying State Space8/2, Discrete Varying State Space1/2
  Discrete Varying State Space1/1 -> Scope WQ/4, To Workspace4/1  "y_q_test_constant1"
  " W selector"/4(Dw) -> Discrete Varying State Space7/5
  " W selector"/1(Aw) -> Discrete Varying State Space7/2
  " W selector"/2(Bw) -> Discrete Varying State Space7/3
  Discrete Varying State Space3/1 -> To Workspace1/1, Measurement Replay Attack2/1(Input2), Scope GH/1  "u_g_test"
  " H selector"/3(Ch) -> Discrete Varying State Space4/4, Discrete Varying State Space2/4
  " H selector"/2(Bh) -> Discrete Varying State Space4/3, Discrete Varying State Space2/3
  " H selector"/4(Dh) -> Discrete Varying State Space4/5, Discrete Varying State Space2/5
  Constant input1/1 -> Discrete Varying State Space3/1, Discrete Varying State Space2/1, To Workspace7/1  "constant_input"
  Discrete Varying State Space4/1 -> To Workspace8/1, Scope GH/3  "u_h_test"
  " H selector"/1(Ah) -> Discrete Varying State Space4/2, Discrete Varying State Space2/2
  Discrete Varying State Space2/1 -> Scope GH/4, To Workspace2/1  "u_h_test_constant"
  " G selector"/4(Dg) -> Discrete Varying State Space3/5
  Measurement Replay Attack2/1(Out2) -> Scope GH/2, Discrete Varying State Space4/1  "~u_g_test"
  " G selector"/2(Bg) -> Discrete Varying State Space3/3
  " G selector"/1(Ag) -> Discrete Varying State Space3/2
  " G selector"/3(Cg) -> Discrete Varying State Space3/4
  Measurement Replay Attack1/1(Out2) -> Discrete Varying State Space8/1, Scope WQ/2  "~y_w_test"

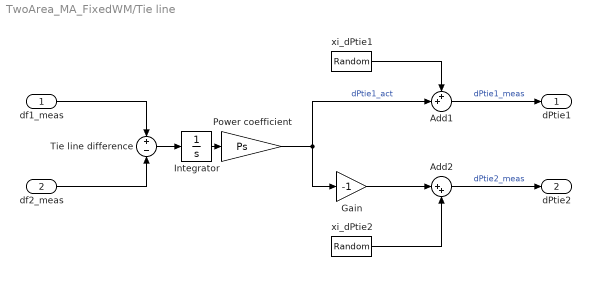
== system TwoArea_MA_FixedWM/Tie line ==
  df1_meas : Inport
  df2_meas : Inport  Port=2
  Add1 : Sum  Inputs=++|
  Add2 : Sum  Inputs=|++
  Gain : Gain  Gain=-1
  Integrator : Integrator
  Power coefficient : Gain  Gain=Ps
  Tie line difference : Sum  Inputs=+-
  xi_dPtie1 : RandomNumber  Variance=xi1.var(2)  Seed=xi1.seeddPtie  SampleTime=0
  xi_dPtie2 : RandomNumber  Variance=xi2.var(2)  Seed=xi2.seeddPtie  SampleTime=0
  dPtie1 : Outport
  dPtie2 : Outport  Port=2
  wires:
  Integrator/1 -> Power coefficient/1
  Power coefficient/1 -> Gain/1, Add1/2  "dPtie1_act"
  xi_dPtie2/1 -> Add2/2
  Gain/1 -> Add2/1
  Add2/1 -> dPtie2/1  "dPtie2_meas"
  Add1/1 -> dPtie1/1  "dPtie1_meas"
  xi_dPtie1/1 -> Add1/1
  df2_meas/1 -> Tie line difference/2
  df1_meas/1 -> Tie line difference/1
  Tie line difference/1 -> Integrator/1

== system TwoArea_MA_FixedWM/W (Watermarker) ==
  y_p : Inport
  " W selector2" : Subsystem
  Demux : Demux  Outputs=3
  Discrete Varying State Space2 : cstblocks/Linear Parameter Varying/Discrete Varying State Space  x0=zeros(wm.N,1)  Ts=ts  OutputX=off  OutputDX=off
      settings: SourceProductBaseCode=CT
  Discrete Varying State Space5 : cstblocks/Linear Parameter Varying/Discrete Varying State Space  x0=zeros(wm.N,1)  Ts=ts  OutputX=off  OutputDX=off
      settings: SourceProductBaseCode=CT
  Discrete Varying State Space6 : cstblocks/Linear Parameter Varying/Discrete Varying State Space  x0=zeros(wm.N,1)  Ts=ts  OutputX=off  OutputDX=off
      settings: SourceProductBaseCode=CT
  Mux4 : Mux  Inputs=3
  W selector 1 : Subsystem
  W selector3 : Subsystem
  y_w : Outport
  wires:
  W selector3/4(Dw) -> Discrete Varying State Space6/5
  " W selector2"/3(Cw) -> Discrete Varying State Space5/4
  " W selector2"/2(Bw) -> Discrete Varying State Space5/3
  " W selector2"/4(Dw) -> Discrete Varying State Space5/5
  Mux4/1 -> y_w/1
  " W selector2"/1(Aw) -> Discrete Varying State Space5/2
  W selector3/3(Cw) -> Discrete Varying State Space6/4
  W selector3/2(Bw) -> Discrete Varying State Space6/3
  Discrete Varying State Space6/1 -> Mux4/3
  Discrete Varying State Space5/1 -> Mux4/2
  W selector3/1(Aw) -> Discrete Varying State Space6/2
  y_p/1 -> Demux/1
  Demux/2 -> Discrete Varying State Space5/1
  Demux/3 -> Discrete Varying State Space6/1
  Demux/1 -> Discrete Varying State Space2/1
  Discrete Varying State Space2/1 -> Mux4/1
  W selector 1/3(Cw) -> Discrete Varying State Space2/4
  W selector 1/1(Aw) -> Discrete Varying State Space2/2
  W selector 1/2(Bw) -> Discrete Varying State Space2/3
  W selector 1/4(Dw) -> Discrete Varying State Space2/5

== system TwoArea_MA_FixedWM/G (Watermarker)/ G selector ==
  Constant10 : Constant  Value=Bg  VectorParams1D=off
  Constant11 : Constant  Value=Cg  VectorParams1D=off
  Constant12 : Constant  Value=Dg  VectorParams1D=off
  Constant9 : Constant  Value=Ag  VectorParams1D=off
  Counter : Subsystem
  MATLAB Function : MATLAB Function  TreatAsAtomicUnit=on
  Ag : Outport
  Bg : Outport  Port=2
  Cg : Outport  Port=3
  Dg : Outport  Port=4
  wires:
  Constant9/1 -> MATLAB Function/2(Aa)
  Constant10/1 -> MATLAB Function/3(Ba)
  Constant11/1 -> MATLAB Function/4(Ca)
  Constant12/1 -> MATLAB Function/5(Da)
  Counter/1(WM_rotation) -> MATLAB Function/1(WM_rotation)
  MATLAB Function/4(D) -> Dg/1
  MATLAB Function/3(C) -> Cg/1
  MATLAB Function/2(B) -> Bg/1
  MATLAB Function/1(A) -> Ag/1

== system TwoArea_MA_FixedWM/G (Watermarker)/ G selector1 ==
  Constant10 : Constant  Value=Bg  VectorParams1D=off
  Constant11 : Constant  Value=Cg  VectorParams1D=off
  Constant12 : Constant  Value=Dg  VectorParams1D=off
  Constant9 : Constant  Value=Ag  VectorParams1D=off
  Counter : Subsystem
  MATLAB Function : MATLAB Function  TreatAsAtomicUnit=on
  Ag : Outport
  Bg : Outport  Port=2
  Cg : Outport  Port=3
  Dg : Outport  Port=4
  wires:
  Constant9/1 -> MATLAB Function/2(Aa)
  Constant10/1 -> MATLAB Function/3(Ba)
  Constant11/1 -> MATLAB Function/4(Ca)
  Constant12/1 -> MATLAB Function/5(Da)
  Counter/1(WM_rotation) -> MATLAB Function/1(WM_rotation)
  MATLAB Function/4(D) -> Dg/1
  MATLAB Function/3(C) -> Cg/1
  MATLAB Function/2(B) -> Bg/1
  MATLAB Function/1(A) -> Ag/1

== system TwoArea_MA_FixedWM/H (Watermark Remover)/ H selector ==
  Constant10 : Constant  Value=Bh  VectorParams1D=off
  Constant11 : Constant  Value=Ch  VectorParams1D=off
  Constant12 : Constant  Value=Dh  VectorParams1D=off
  Constant9 : Constant  Value=Ah  VectorParams1D=off
  Counter : Subsystem
  MATLAB Function : MATLAB Function  TreatAsAtomicUnit=on
  Ah : Outport
  Bh : Outport  Port=2
  Ch : Outport  Port=3
  Dh : Outport  Port=4
  wires:
  Constant9/1 -> MATLAB Function/2(Aa)
  Constant10/1 -> MATLAB Function/3(Ba)
  Constant11/1 -> MATLAB Function/4(Ca)
  Constant12/1 -> MATLAB Function/5(Da)
  Counter/1(WM_rotation) -> MATLAB Function/1(WM_rotation)
  MATLAB Function/4(D) -> Dh/1
  MATLAB Function/3(C) -> Ch/1
  MATLAB Function/2(B) -> Bh/1
  MATLAB Function/1(A) -> Ah/1

== system TwoArea_MA_FixedWM/H (Watermark Remover)/ H selector1 ==
  Constant10 : Constant  Value=Bh  VectorParams1D=off
  Constant11 : Constant  Value=Ch  VectorParams1D=off
  Constant12 : Constant  Value=Dh  VectorParams1D=off
  Constant9 : Constant  Value=Ah  VectorParams1D=off
  Counter : Subsystem
  MATLAB Function : MATLAB Function  TreatAsAtomicUnit=on
  Ah : Outport
  Bh : Outport  Port=2
  Ch : Outport  Port=3
  Dh : Outport  Port=4
  wires:
  Constant9/1 -> MATLAB Function/2(Aa)
  Constant10/1 -> MATLAB Function/3(Ba)
  Constant11/1 -> MATLAB Function/4(Ca)
  Constant12/1 -> MATLAB Function/5(Da)
  Counter/1(WM_rotation) -> MATLAB Function/1(WM_rotation)
  MATLAB Function/4(D) -> Dh/1
  MATLAB Function/3(C) -> Ch/1
  MATLAB Function/2(B) -> Bh/1
  MATLAB Function/1(A) -> Ah/1

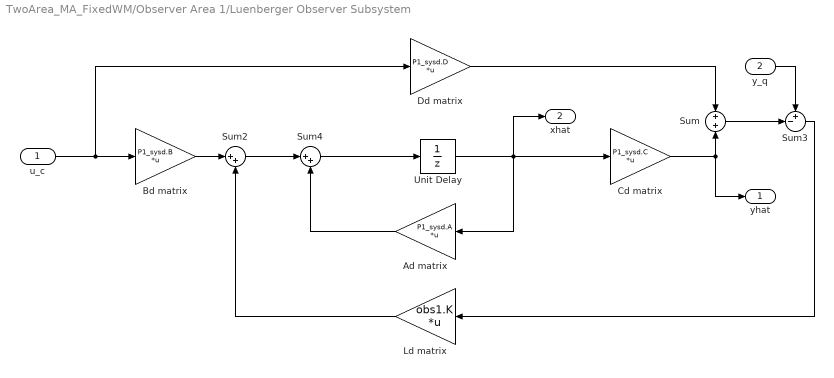
== system TwoArea_MA_FixedWM/Observer Area 1/Luenberger Observer Subsystem ==
  u_c : Inport
  y_q : Inport  Port=2
  Ad matrix : Gain  Gain=P1_sysd.A  Multiplication=Matrix(K*u)
  Bd matrix : Gain  Gain=P1_sysd.B  Multiplication=Matrix(K*u)
  Cd matrix : Gain  Gain=P1_sysd.C  Multiplication=Matrix(K*u)
  Dd matrix : Gain  Gain=P1_sysd.D  Multiplication=Matrix(K*u)
  Ld matrix : Gain  Gain=obs1.K  Multiplication=Matrix(K*u)
  Sum : Sum
  Sum2 : Sum  Inputs=|++
  Sum3 : Sum  Inputs=+-|
  Sum4 : Sum  Inputs=|++
  Unit Delay : UnitDelay  InitialCondition=obs1.x_hat0  SampleTime=ts  HasFrameUpgradeWarning=on
  yhat : Outport
  xhat : Outport  Port=2  VectorParamsAs1DForOutWhenUnconnected=off
  wires:
  Dd matrix/1 -> Sum/1
  Sum2/1 -> Sum4/1
  Sum3/1 -> Ld matrix/1
  Unit Delay/1 -> xhat/1, Ad matrix/1, Cd matrix/1
  u_c/1 -> Bd matrix/1, Dd matrix/1
  Sum4/1 -> Unit Delay/1
  Bd matrix/1 -> Sum2/1
  Ld matrix/1 -> Sum2/2
  Cd matrix/1 -> Sum/2, yhat/1
  Ad matrix/1 -> Sum4/2
  y_q/1 -> Sum3/1
  Sum/1 -> Sum3/2

== system TwoArea_MA_FixedWM/Q (Watermark Remover)/ Q selector ==
  Constant10 : Constant  Value=Bq  VectorParams1D=off
  Constant11 : Constant  Value=Cq  VectorParams1D=off
  Constant12 : Constant  Value=Dq  VectorParams1D=off
  Constant9 : Constant  Value=Aq  VectorParams1D=off
  Counter : Subsystem
  MATLAB Function : MATLAB Function  TreatAsAtomicUnit=on
  Aq : Outport
  Bq : Outport  Port=2
  Cq : Outport  Port=3
  Dq : Outport  Port=4
  wires:
  Constant9/1 -> MATLAB Function/2(Aa)
  Constant10/1 -> MATLAB Function/3(Ba)
  Constant11/1 -> MATLAB Function/4(Ca)
  Constant12/1 -> MATLAB Function/5(Da)
  Counter/1(WM_rotation) -> MATLAB Function/1(WM_rotation)
  MATLAB Function/4(D) -> Dq/1
  MATLAB Function/3(C) -> Cq/1
  MATLAB Function/2(B) -> Bq/1
  MATLAB Function/1(A) -> Aq/1

== system TwoArea_MA_FixedWM/Q (Watermark Remover)/ Q selector1 ==
  Constant10 : Constant  Value=Bq  VectorParams1D=off
  Constant11 : Constant  Value=Cq  VectorParams1D=off
  Constant12 : Constant  Value=Dq  VectorParams1D=off
  Constant9 : Constant  Value=Aq  VectorParams1D=off
  Counter : Subsystem
  MATLAB Function : MATLAB Function  TreatAsAtomicUnit=on
  Aq : Outport
  Bq : Outport  Port=2
  Cq : Outport  Port=3
  Dq : Outport  Port=4
  wires:
  Constant9/1 -> MATLAB Function/2(Aa)
  Constant10/1 -> MATLAB Function/3(Ba)
  Constant11/1 -> MATLAB Function/4(Ca)
  Constant12/1 -> MATLAB Function/5(Da)
  Counter/1(WM_rotation) -> MATLAB Function/1(WM_rotation)
  MATLAB Function/4(D) -> Dq/1
  MATLAB Function/3(C) -> Cq/1
  MATLAB Function/2(B) -> Bq/1
  MATLAB Function/1(A) -> Aq/1

== system TwoArea_MA_FixedWM/Q (Watermark Remover)/ Q selector2 ==
  Constant10 : Constant  Value=Bq  VectorParams1D=off
  Constant11 : Constant  Value=Cq  VectorParams1D=off
  Constant12 : Constant  Value=Dq  VectorParams1D=off
  Constant9 : Constant  Value=Aq  VectorParams1D=off
  Counter : Subsystem
  MATLAB Function : MATLAB Function  TreatAsAtomicUnit=on
  Aq : Outport
  Bq : Outport  Port=2
  Cq : Outport  Port=3
  Dq : Outport  Port=4
  wires:
  Constant9/1 -> MATLAB Function/2(Aa)
  Constant10/1 -> MATLAB Function/3(Ba)
  Constant11/1 -> MATLAB Function/4(Ca)
  Constant12/1 -> MATLAB Function/5(Da)
  Counter/1(WM_rotation) -> MATLAB Function/1(WM_rotation)
  MATLAB Function/4(D) -> Dq/1
  MATLAB Function/3(C) -> Cq/1
  MATLAB Function/2(B) -> Bq/1
  MATLAB Function/1(A) -> Aq/1

== system TwoArea_MA_FixedWM/Simple Cyber-Attack/Cyber-attack control commands ==
  In1 : Inport
  Add14 : Sum
  Gain : Gain  Gain=ca.at1
  Multiport Switch : MultiPortSwitch  InputSameDT=on
  Random Source : dspsrcs4/Random Source  SrcType=Uniform  NormMethod=Ziggurat  CltLength=12  MinVal=0  MaxVal=ca.at2  MeanVal=0  VarVal=1  RepMode=Not repeatable  rawSeed=1  IsInherit=off  SampMode=Discrete  SampTime=1  SampFrame=1  DataType=Double  OutComplex=Real  OutputFrames=off
  Step : Step  Time=attack_start  Before=1  After=attack_type  SampleTime=0
  Out1 : Outport
  wires:
  In1/1 -> Add14/1, Gain/1, Multiport Switch/2
  Random Source/1 -> Add14/2
  Gain/1 -> Multiport Switch/3
  Add14/1 -> Multiport Switch/4
  Step/1 -> Multiport Switch/1
  Multiport Switch/1 -> Out1/1

== system TwoArea_MA_FixedWM/Simple Cyber-Attack/Cyber-attack measurements ==
  In1 : Inport
  Add14 : Sum
  Gain : Gain  Gain=ca.at1
  Multiport Switch : MultiPortSwitch  InputSameDT=on
  Random Source : dspsrcs4/Random Source  SrcType=Uniform  NormMethod=Ziggurat  CltLength=12  MinVal=0  MaxVal=ca.at2  MeanVal=0  VarVal=1  RepMode=Not repeatable  rawSeed=1  IsInherit=off  SampMode=Discrete  SampTime=1  SampFrame=1  DataType=Double  OutComplex=Real  OutputFrames=off
  Step : Step  Time=attack_start  Before=1  After=attack_type  SampleTime=0
  Out1 : Outport
  wires:
  In1/1 -> Gain/1, Add14/1, Multiport Switch/2
  Random Source/1 -> Add14/2
  Add14/1 -> Multiport Switch/4
  Step/1 -> Multiport Switch/1
  Multiport Switch/1 -> Out1/1
  Gain/1 -> Multiport Switch/3

== system TwoArea_MA_FixedWM/Testing Watermarking/ G selector ==
  Constant10 : Constant  Value=Bg  VectorParams1D=off
  Constant11 : Constant  Value=Cg  VectorParams1D=off
  Constant12 : Constant  Value=Dg  VectorParams1D=off
  Constant9 : Constant  Value=Ag  VectorParams1D=off
  Counter : Subsystem
  MATLAB Function : MATLAB Function  TreatAsAtomicUnit=on
  Ag : Outport
  Bg : Outport  Port=2
  Cg : Outport  Port=3
  Dg : Outport  Port=4
  wires:
  Constant9/1 -> MATLAB Function/2(Aa)
  Constant10/1 -> MATLAB Function/3(Ba)
  Constant11/1 -> MATLAB Function/4(Ca)
  Constant12/1 -> MATLAB Function/5(Da)
  Counter/1(WM_rotation) -> MATLAB Function/1(WM_rotation)
  MATLAB Function/4(D) -> Dg/1
  MATLAB Function/3(C) -> Cg/1
  MATLAB Function/2(B) -> Bg/1
  MATLAB Function/1(A) -> Ag/1

== system TwoArea_MA_FixedWM/Testing Watermarking/ H selector ==
  Constant10 : Constant  Value=Bh  VectorParams1D=off
  Constant11 : Constant  Value=Ch  VectorParams1D=off
  Constant12 : Constant  Value=Dh  VectorParams1D=off
  Constant9 : Constant  Value=Ah  VectorParams1D=off
  Counter : Subsystem
  MATLAB Function : MATLAB Function  TreatAsAtomicUnit=on
  Ah : Outport
  Bh : Outport  Port=2
  Ch : Outport  Port=3
  Dh : Outport  Port=4
  wires:
  Constant9/1 -> MATLAB Function/2(Aa)
  Constant10/1 -> MATLAB Function/3(Ba)
  Constant11/1 -> MATLAB Function/4(Ca)
  Constant12/1 -> MATLAB Function/5(Da)
  Counter/1(WM_rotation) -> MATLAB Function/1(WM_rotation)
  MATLAB Function/4(D) -> Dh/1
  MATLAB Function/3(C) -> Ch/1
  MATLAB Function/2(B) -> Bh/1
  MATLAB Function/1(A) -> Ah/1

== system TwoArea_MA_FixedWM/Testing Watermarking/ Q selector ==
  Constant10 : Constant  Value=Bq  VectorParams1D=off
  Constant11 : Constant  Value=Cq  VectorParams1D=off
  Constant12 : Constant  Value=Dq  VectorParams1D=off
  Constant9 : Constant  Value=Aq  VectorParams1D=off
  Counter : Subsystem
  MATLAB Function : MATLAB Function  TreatAsAtomicUnit=on
  Aq : Outport
  Bq : Outport  Port=2
  Cq : Outport  Port=3
  Dq : Outport  Port=4
  wires:
  Constant9/1 -> MATLAB Function/2(Aa)
  Constant10/1 -> MATLAB Function/3(Ba)
  Constant11/1 -> MATLAB Function/4(Ca)
  Constant12/1 -> MATLAB Function/5(Da)
  Counter/1(WM_rotation) -> MATLAB Function/1(WM_rotation)
  MATLAB Function/4(D) -> Dq/1
  MATLAB Function/3(C) -> Cq/1
  MATLAB Function/2(B) -> Bq/1
  MATLAB Function/1(A) -> Aq/1

== system TwoArea_MA_FixedWM/Testing Watermarking/ W selector ==
  Constant10 : Constant  Value=Bw  VectorParams1D=off
  Constant11 : Constant  Value=Cw  VectorParams1D=off
  Constant12 : Constant  Value=Dw  VectorParams1D=off
  Constant9 : Constant  Value=Aw  VectorParams1D=off
  Counter : Subsystem
  MATLAB Function : MATLAB Function  TreatAsAtomicUnit=on
  Aw : Outport
  Bw : Outport  Port=2
  Cw : Outport  Port=3
  Dw : Outport  Port=4
  wires:
  Constant9/1 -> MATLAB Function/2(Aa)
  Constant10/1 -> MATLAB Function/3(Ba)
  Constant11/1 -> MATLAB Function/4(Ca)
  Constant12/1 -> MATLAB Function/5(Da)
  Counter/1(WM_rotation) -> MATLAB Function/1(WM_rotation)
  MATLAB Function/4(D) -> Dw/1
  MATLAB Function/3(C) -> Cw/1
  MATLAB Function/2(B) -> Bw/1
  MATLAB Function/1(A) -> Aw/1

== system TwoArea_MA_FixedWM/Testing Watermarking/Cyber-attack measurements ==
  In1 : Inport
  Add10 : Sum  Commented=on
  Add14 : Sum
  Clock : Clock  Commented=on
  Constant : Constant  Commented=on  Value=attack_start
  Gain : Gain  Gain=2
  Gain1 : Gain  Commented=on  Gain=ca.at1
  Multiport Switch : MultiPortSwitch  InputSameDT=on
  Random Source : dspsrcs4/Random Source  SrcType=Uniform  NormMethod=Ziggurat  CltLength=12  MinVal=0  MaxVal=ca.at2  MeanVal=0  VarVal=1  RepMode=Not repeatable  rawSeed=1  IsInherit=off  SampMode=Discrete  SampTime=1  SampFrame=1  DataType=Double  OutComplex=Real  OutputFrames=off
  Step : Step  Time=attack_start  Before=1  After=attack_type  SampleTime=0
  Sum : Sum  Commented=on  Inputs=-+
  Out1 : Outport
  wires:
  In1/1 -> Gain/1, Add14/1, Multiport Switch/2
  Random Source/1 -> Add14/2
  Add14/1 -> Multiport Switch/4
  Step/1 -> Multiport Switch/1
  Multiport Switch/1 -> Out1/1
  Clock/1 -> Sum/2
  Sum/1 -> Gain1/1
  Gain1/1 -> Add10/2
  ? -> Add10/1
  Add10/1 -> ?
  Constant/1 -> Sum/1
  Gain/1 -> Multiport Switch/3

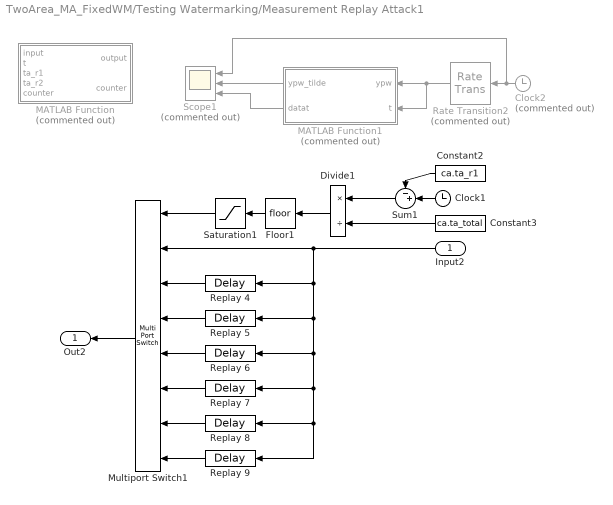
== system TwoArea_MA_FixedWM/Testing Watermarking/Measurement Replay Attack1 ==
  Input2 : Inport
  Clock1 : Clock
  Clock2 : Clock  Commented=on
  Constant2 : Constant  Value=ca.ta_r1
  Constant3 : Constant  Value=ca.ta_total
  Divide1 : Product  Inputs=*/  OutMin=0  OutMax=3  SaturateOnIntegerOverflow=on
  Floor1 : Rounding
  MATLAB Function : MATLAB Function  Commented=on  TreatAsAtomicUnit=on
  MATLAB Function1 : MATLAB Function  Commented=on  TreatAsAtomicUnit=on
  Multiport Switch1 : MultiPortSwitch  DataPortOrder=Zero-based contiguous  Inputs=7  zeroidx=on
  Rate Transition2 : RateTransition  Commented=on  OutPortSampleTime=1
  Replay 4 : TransportDelay  DelayTime=ca.ta_total
  Replay 5 : TransportDelay  DelayTime=ca.ta_total*2
  Replay 6 : TransportDelay  DelayTime=ca.ta_total*3
  Replay 7 : TransportDelay  DelayTime=ca.ta_total*4
  Replay 8 : TransportDelay  DelayTime=ca.ta_total*5
  Replay 9 : TransportDelay  DelayTime=ca.ta_total*6
  Saturation1 : Saturate  UpperLimit=6  LowerLimit=0
  Scope1 : Scope  Commented=on  NumInputPorts=3
  Sum1 : Sum  Inputs=-+|
  Out2 : Outport
  wires:
  Replay 7/1 -> Multiport Switch1/6
  Replay 8/1 -> Multiport Switch1/7
  Replay 9/1 -> Multiport Switch1/8
  Divide1/1 -> Floor1/1
  Clock1/1 -> Sum1/2
  Constant2/1 -> Sum1/1
  Replay 5/1 -> Multiport Switch1/4
  Multiport Switch1/1 -> Out2/1
  Constant3/1 -> Divide1/2
  Replay 6/1 -> Multiport Switch1/5
  Floor1/1 -> Saturation1/1
  Input2/1 -> Replay 9/1, Replay 8/1, Replay 7/1, Replay 6/1, Replay 5/1, Replay 4/1, Multiport Switch1/2
  Sum1/1 -> Divide1/1
  Saturation1/1 -> Multiport Switch1/1
  Replay 4/1 -> Multiport Switch1/3
  Rate Transition2/1 -> MATLAB Function1/2(t), MATLAB Function1/1(ypw)
  Clock2/1 -> Scope1/1, Rate Transition2/1
  MATLAB Function1/2(datat) -> Scope1/3
  MATLAB Function1/1(ypw_tilde) -> Scope1/2
